simulink model "riccati"  (R2016b)
settings: Solver=FixedStepAuto  StartTime=0.0  StopTime=T  FixedStep=stepsize  RelTol=1e-3
values from neighbouring files (symbols this model uses):
  A = [0.2 0.7 ... (first row only)    [main.m]
  B = [0.1 0.5]'    [main.m]
  M = lyap(Abar',Q+k'*R*k)    [main.m]
  Q = eye(2)    [main.m]
  R = eye(1)    [main.m]
settings Model: Creator=Berk  LastModifiedBy=Berk

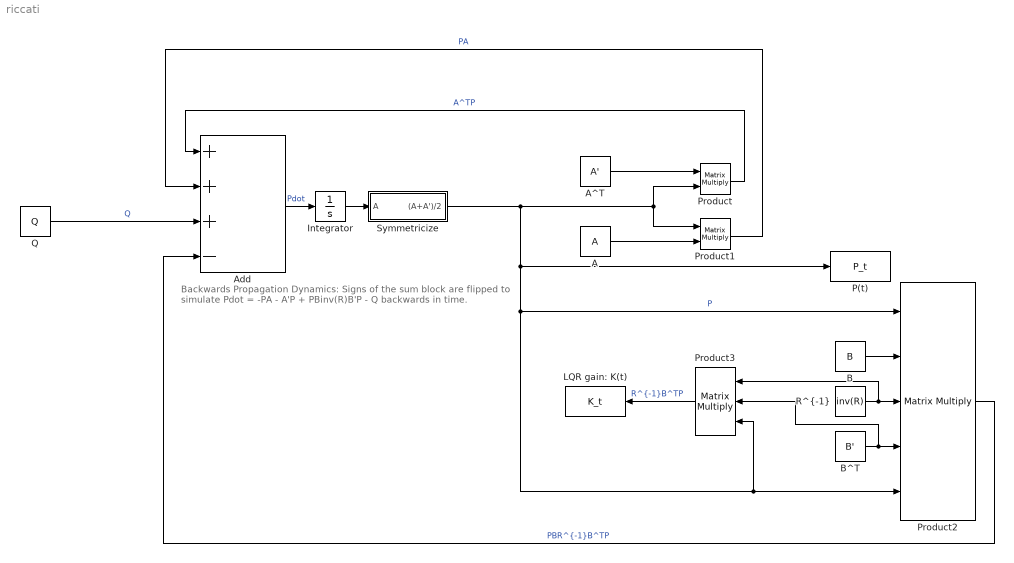
== system riccati ==
  note: Backwards Propagation Dynamics: Signs of the sum block are flipped to simulate Pdot = -PA - A'P + PBinv(R)B'P - Q backwards in time.
  A : Constant  Value=A  VectorParams1D=off
  A^T : Constant  Value=A'  VectorParams1D=off
  Add : Sum  Inputs=+++-
  B : Constant  Value=B  VectorParams1D=off
  B^T : Constant  Value=B'  VectorParams1D=off
  Integrator : Integrator  InitialCondition=M
  LQR gain: K(t) : ToWorkspace  VariableName=K_t  SaveFormat=Timeseries  SampleTime=-1
  P(t) : ToWorkspace  VariableName=P_t  SaveFormat=Timeseries  SampleTime=-1
  Product : Product  Multiplication=Matrix(*)
  Product1 : Product  Multiplication=Matrix(*)
  Product2 : Product  Inputs=5  Multiplication=Matrix(*)
  Product3 : Product  Inputs=3  Multiplication=Matrix(*)
  Q : Constant  Value=Q  VectorParams1D=off
  "R^{-1}" : Constant  Value=inv(R)  VectorParams1D=off
  Symmetricize : Subsystem
  wires:
  A^T/1 -> Product/1
  A/1 -> Product1/2
  Product/1 -> Add/1  "A^TP"
  Product1/1 -> Add/2  "PA"
  Add/1 -> Integrator/1  "Pdot"
  Symmetricize/1((A+A')/2) -> Product3/3, Product2/5, Product2/1, P(t)/1, Product1/1, Product/2  "P"
  B/1 -> Product2/2
  Q/1 -> Add/3  "Q"
  Product2/1 -> Add/4  "PBR^{-1}B^TP"
  "R^{-1}"/1 -> Product3/1, Product2/3
  B^T/1 -> Product3/2, Product2/4
  Product3/1 -> LQR gain: K(t)/1  "R^{-1}B^TP"
  Integrator/1 -> Symmetricize/1(A)

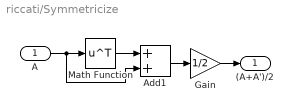
== system riccati/Symmetricize ==
  A : Inport
  Add1 : Sum
  Gain : Gain  Gain=1/2
  Math Function : Math  Operator=transpose  SaturateOnIntegerOverflow=on
  (A+A')/2 : Outport
  wires:
  Math Function/1 -> Add1/1
  Gain/1 -> (A+A')/2/1
  A/1 -> Add1/2, Math Function/1
  Add1/1 -> Gain/1
